simulink model "VVVF_control"  (R2018b)
settings: Solver=ode23tb  StartTime=0.0  StopTime=3  RelTol=1e-3  EnableMultiTasking=on
libraries: powerlib x8, powerlib_meascontrol x1, powerlib_extras x1
settings Model: Creator=Administrator  LastModifiedBy=13646769405
settings DataIOCC: LimitDataPoints=on  SaveFormat=Array  SignalLoggingSaveFormat=ModelDataLogs
settings OptimizationCC: ExpressionDepthLimit=2147483647  LifeSpan=inf
settings DebuggingCC: UnderspecifiedInitializationDetection=Classic  MergeDetectMultiDrivingBlocksExec=none  SolverPrmCheckMsg=warning  FcnCallInpInsideContextMsg=warning  StateNameClashWarn=warning  SFUnexpectedBacktrackingDiag=warning  SFNoUnconditionalDefaultTransitionDiag=warning  SFExecutionAtInitializationDiag=none
settings HardwareCC: ProdBitPerPointer=32  ProdBitPerSizeT=32  ProdBitPerPtrDiffT=32  ProdLargestAtomicFloat=None  ProdIntDivRoundTo=Undefined  ProdEndianess=Unspecified  ProdWordSize=32  ProdHWDeviceType=32-bit Generic
settings ModelReferenceCC: PropagateSignalLabelsOutOfModel=off
settings SFSimCC: SimUseLocalCustomCode=off
settings RTWCC: RTWUseLocalCustomCode=off
settings CodeAppCC: StateflowObjectComments=on
settings GRTTargetCC: TargetLangStandard=C89/C90 (ANSI)  GeneratePreprocessorConditionals=Disable all
settings ConfigComp: CovMetricSettings=dw  CovHtmlReporting=on  CovSaveCumulativeToWorkspaceVar=on  CovSaveSingleToWorkspaceVar=on  CovExternalEMLEnable=off
settings SimscapeCC: SimscapeNormalizeSystem=off

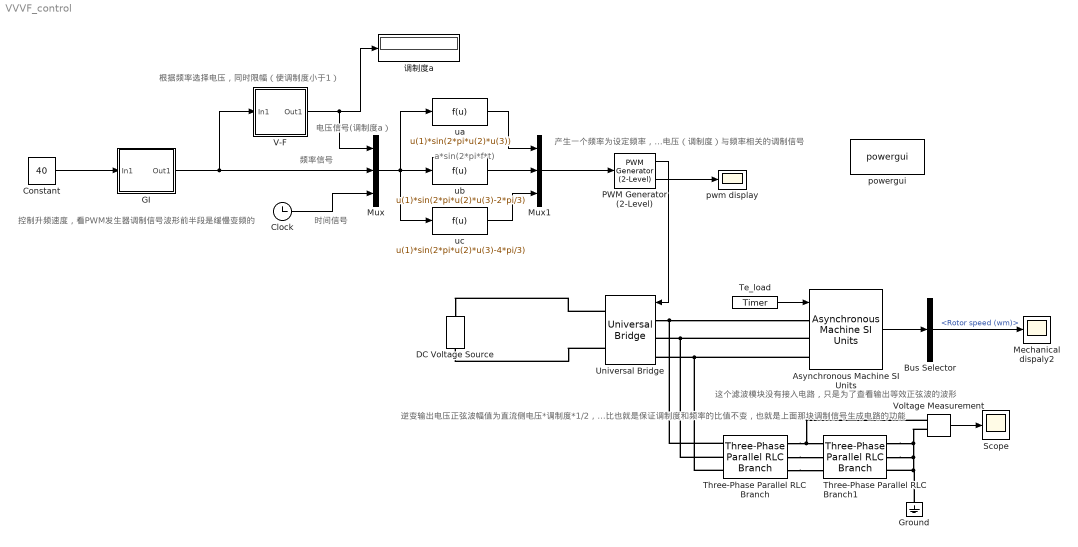
== system VVVF_control ==
  note: 这个滤波模块没有接入电路，只是为了查看输出等效正弦波的波形
  note: a*sin(2*pi*f*t)
  note: 逆变输出电压正弦波幅值为直流侧电压*调制度*1/2，他正比于调制度，所以恒压频比也就是保证调制度和频率的比值不变，也就是上面那块调制信号生成电路的功能
  note: 产生一个频率为设定频率，电压（调制度）与频率相关的调制信号
  note: 时间信号
  note: 频率信号
  note: 电压信号(调制度a）
  note: 根据频率选择电压，同时限幅（使调制度小于1）
  note: 控制升频速度，看PWM发生器调制信号波形前半段是缓慢变频的
  Asynchronous Machine SI Units : powerlib/Machines/Asynchronous Machine SI Units  RotorType=Squirrel-cage  PresetModel=No  MechanicalLoad=Torque Tm  ShowDetailedParameters=on  ReferenceFrame=Rotor  Units=SI  MeasurementBus=off  NominalParameters=[ 2200, 380, 50 ]  Stator=[ 3.478 0.01254]  Rotor=[ 2.546 0.01226]  Cage1=[ 0.022 0.226/377]  Cage2=[ 0.022 0.226/377]  Lm=0.3329  Mechanical="[ 0.0131  0  2 ]"  PolePairs=2  InitialConditions=[1 0 0 0 0 0 0 0]  SimulateSaturation=off  Saturation=[14.03593122, 27.81365428, 53.79336849, 72.68890987, 97.98006896, 148.6815601, 215.7428561, 302.9841135, 420.4778367 ; 230, 322, 414, 460, 506, 552, 598, 644, 690]  LoadFlowParameters=1492000  TsPowergui=0  TsBlock=-1  IterativeModel=Forward Euler  IterativeDiscreteModel=Trapezoidal non iterative  Pmec=0
      settings: SourceProductName=Simscape Electrical
  Bus Selector : BusSelector  OutputSignals=Mechanical.Rotor speed (wm)
  Clock : Clock
  Constant : Constant  Value=40
  DC Voltage Source : powerlib/Electrical Sources/DC Voltage Source  Amplitude=514  Measurements=None
      settings: SourceProductName=Simscape Electrical
  GI : Subsystem
  Ground : powerlib/Elements/Ground  LConnTagsString=a
      settings: SourceProductName=Simscape Electrical
  Mechanical dispaly2 : Scope
  Mux : Mux  Inputs=3
  Mux1 : Mux  Inputs=3
  PWM Generator (2-Level) : powerlib_meascontrol/Pulse & Signal Generators/PWM Generator (2-Level)  ModulatorType=Three-phase bridge (6 pulses)  ModulatorMode=Unsynchronized  Fc=10000  Pc=0  nF=27  MinMax="[ -1  1 ]"  SamplingTechnique=Natural  ModulatingSignals=off  m=0.8  Freq=60  Phase=0  Ts=0  ShowCarrierOutport=on
  Scope : Scope
  Te_load : powerlib_extras/Control  Blocks/Timer  t="[ 0  0.5  4  ]"  e="[0  14.764 14.764]"
  Three-Phase Parallel RLC Branch : powerlib/Elements/Three-Phase Parallel RLC Branch  LConnTagsString=A|B|C  RConnTagsString=A|B|C  BranchType=R  Resistance=1e3  Inductance=1e-3  Capacitance=1e-6  Measurements=None
      settings: SourceProductName=Simscape Electrical  SourceProductBaseCode=PS
  Three-Phase Parallel RLC Branch1 : powerlib/Elements/Three-Phase Parallel RLC Branch  LConnTagsString=A|B|C  RConnTagsString=A|B|C  BranchType=C  Resistance=1  Inductance=1e-3  Capacitance=1e-6  Measurements=None
      settings: SourceProductName=Simscape Electrical  SourceProductBaseCode=PS
  Universal Bridge : powerlib/Power Electronics/Universal Bridge  Arms=3  SnubberResistance=1e5  SnubberCapacitance=inf  Device=IGBT / Diodes  Ron=1e-3  Lon=0  ForwardVoltages="[  0  0  ]"  ForwardVoltage=0  GTOparameters=[ 10e-6 , 20e-6 ]  IGBTparameters=[ 1e-6 , 2e-6 ]  Measurements=None  Measurements_2=None  converterType=Rectifier
      settings: SourceProductName=Simscape Electrical
  V-F : Subsystem
  Voltage Measurement : powerlib/Measurements/Voltage Measurement  PhasorSimulation=off  OutputType=Complex  PSBequivalent=0
      settings: SourceProductName=Simscape Electrical
  powergui : powerlib/powergui  Priority=1  SimulationMode=Continuous  SampleTime=50e-6  frequency=60  Iterations=50  frequencyindice=50  Pbase=100e6  ErrMax=1e-4  UnitsV=kV  UnitsW=MW  buscounter=0  FunctionMessages=off  echomessages=off  EnableUseOfTLC=off  CurrentSourceSwitches=off  DisableSnubberDevices=off  DisableRonSwitches=off  DisableVfSwitches=off  DisplayEquations=off  SolverType=Tustin/Backward Euler (TBE)  Interpol=off  ExternalGateDelay=off  methode=off  Ts=100  x0status=blocks  SPID=on  SwTol=0  HookPort=off  RestoreLinks=warning  ResistiveCurrentMeasurement=off  Frange=[0:2:500]  Ylog=off  Xlog=on  ShowGrid=off  save=off  variable=ZData  structure=0  ZoomFFT=off  StartTime=0.0  cycles=1  DisplayStyle=1  fundamental=60  FreqAxis=off  MaxFrequency=1000  frequencyindicesteady=1  RmsSteady=1  display=off
  pwm display : Scope
  ua : Fcn  Expr=u(1)*sin(2*pi*u(2)*u(3))
  ub : Fcn  Expr=u(1)*sin(2*pi*u(2)*u(3)-2*pi/3)
  uc : Fcn  Expr=u(1)*sin(2*pi*u(2)*u(3)-4*pi/3)
  调制度a : Display
  wires:
  Te_load/1 -> Asynchronous Machine SI Units/1
  Asynchronous Machine SI Units/1 -> Bus Selector/1
  Bus Selector/1 -> Mechanical dispaly2/1  "<Rotor speed (wm)>"
  GI/1(Out1) -> V-F/1(In1), Mux/2
  Constant/1 -> GI/1(In1)
  Clock/1 -> Mux/3
  V-F/1(Out1) -> Mux/1, 调制度a/1
  Mux/1 -> ua/1, uc/1, ub/1
  ua/1 -> Mux1/1
  ub/1 -> Mux1/2
  uc/1 -> Mux1/3
  Mux1/1 -> PWM Generator (2-Level)/1
  PWM Generator (2-Level)/2 -> pwm display/1
  PWM Generator (2-Level)/1 -> Universal Bridge/1
  Voltage Measurement/1 -> Scope/1
  connections:
  Universal Bridge/LConn1 -- Three-Phase Parallel RLC Branch/LConn1 -- Asynchronous Machine SI Units/LConn1
  Asynchronous Machine SI Units/LConn2 -- Three-Phase Parallel RLC Branch/LConn2 -- Universal Bridge/LConn2
  Asynchronous Machine SI Units/LConn3 -- Three-Phase Parallel RLC Branch/LConn3 -- Universal Bridge/LConn3
  Universal Bridge/RConn2 -- DC Voltage Source/LConn1
  Universal Bridge/RConn1 -- DC Voltage Source/RConn1
  Three-Phase Parallel RLC Branch1/RConn1 -- Voltage Measurement/LConn2 -- Three-Phase Parallel RLC Branch1/RConn2 -- Ground/LConn1 -- Three-Phase Parallel RLC Branch1/RConn3
  Three-Phase Parallel RLC Branch/RConn1 -- Voltage Measurement/LConn1 -- Three-Phase Parallel RLC Branch1/LConn1
  Three-Phase Parallel RLC Branch/RConn2 -- Three-Phase Parallel RLC Branch1/LConn2
  Three-Phase Parallel RLC Branch/RConn3 -- Three-Phase Parallel RLC Branch1/LConn3

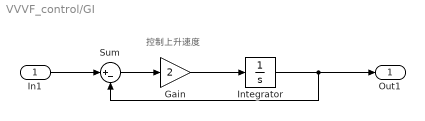
== system VVVF_control/GI ==
  note: 控制上升速度
  In1 : Inport
  Gain : Gain  Gain=2
  Integrator : Integrator
  Sum : Sum  Inputs=|+-
  Out1 : Outport
  wires:
  Integrator/1 -> Out1/1, Sum/2
  Gain/1 -> Integrator/1
  In1/1 -> Sum/1
  Sum/1 -> Gain/1

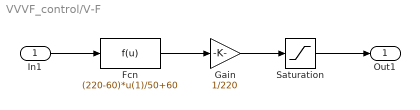
== system VVVF_control/V-F ==
  In1 : Inport
  Fcn : Fcn  Expr=(220-60)*u(1)/50+60
  Gain : Gain  Gain=1/220
  Saturation : Saturate  UpperLimit=0.95  LowerLimit=-0.95
  Out1 : Outport
  wires:
  Fcn/1 -> Gain/1
  In1/1 -> Fcn/1
  Gain/1 -> Saturation/1
  Saturation/1 -> Out1/1
